simulink model "GridFormingConverter"  (R2024b)
settings: Solver=ode1be  StartTime=0.0  StopTime=simulationTime  FixedStep=gridInverter.vsm.samplingTime  MaxStep=gridInverter.vsm.samplingTime  RelTol=1e-3  AbsTol=1e-3
PreLoadFcn:
  | % Parameterize the model
  | GridFormingConverterInputParameters;
  | GFLParameters;
PostLoadFcn:
  | GridFormingConverterTestCondition;
  | GFLParameters;
undefined symbols (not defined in the file or in its folder): base, ConvCtrl, ConvPlt, DiscIntNeverNeededParam, Discrete, Fault, gcbh, GFMGFLSelect, grid, gridInverter, HMI, localSolverSampleTime, magnitude, PlantSim, scrFactorRg, scrFactorXg, sps, sps_rtmsupport, spsPLL3phModel, transformer, TransmissionLine, Trf
libraries: powerlib_extras x39, ee_lib x21, eeGeneralControl x19, nesl_utility x16, simulink x13, eeTransforms x10, fl_lib x7, spsSecondOrderFilterLib x4, spsabctodq0Lib x4, spsPower3phInstantaneousLib x3, spsMeanLib x2, eeSinGeneratorThreePhase x1
(part 3 of 6)

== system GridFormingConverter/BusCalculations/Measurement Unit (Phasor Computation)/Discrete Fourier(A) ==
  note: Discrete Fourier
  note: Pierre Giroux, Gilbert Sybille
      | Power System Simulation Laboratory
      | IREQ, Hydro-Quebc
  In : Inport
  Demux : Demux  Outputs=2
      settings: DisplayOption=none
  Discrete Mean value1 : powerlib_extras/Discrete Measurements/Discrete  Mean value  Freq=Freq  Vinit=Real_Init  Ts=Ts
  Discrete Mean value2 : powerlib_extras/Discrete Measurements/Discrete  Mean value  Freq=Freq  Vinit=Imag_Init  Ts=Ts
  Gain : Gain  Gain=2*pi*n*Freq  SaturateOnIntegerOverflow=on  OutDataTypeStr=Inherit: Same as input  ParamDataTypeStr=Inherit: Same as input
  Gain1 : Gain  Gain=k  SaturateOnIntegerOverflow=on  OutDataTypeStr=Inherit: Same as input  ParamDataTypeStr=Inherit: Same as input
  Mux : Mux  Inputs=2
  Product : Product  InputSameDT=on  SaturateOnIntegerOverflow=on  OutDataTypeStr=Inherit: Same as first input
  Real-Imag to Complex : RealImagToComplex
  Trigonometric Function : Trigonometry
  Trigonometric Function1 : Trigonometry  Operator=cos
  t : DigitalClock  SampleTime=Ts
  Fund : Outport
  wires:
  Real-Imag to Complex/1 -> Fund/1
  Discrete Mean value2/1 -> Real-Imag to Complex/2  "Imag"
  Discrete Mean value1/1 -> Real-Imag to Complex/1  "Real"
  t/1 -> Gain/1
  Gain/1 -> Trigonometric Function/1, Trigonometric Function1/1
  Trigonometric Function/1 -> Mux/1
  Trigonometric Function1/1 -> Mux/2
  Mux/1 -> Gain1/1
  In/1 -> Product/1
  Gain1/1 -> Product/2
  Product/1 -> Demux/1
  Demux/1 -> Discrete Mean value1/1
  Demux/2 -> Discrete Mean value2/1

== system GridFormingConverter/BusCalculations/Measurement Unit (Phasor Computation)/Discrete Fourier(A)  ==
  note: Pierre Giroux, Gilbert Sybille
      | Power System Simulation Laboratory
      | IREQ, Hydro-Quebc
  note: Discrete Fourier
  In : Inport
  Demux : Demux  Outputs=2
      settings: DisplayOption=none
  Discrete Mean value1 : powerlib_extras/Discrete Measurements/Discrete  Mean value  Freq=Freq  Vinit=Real_Init  Ts=Ts
  Discrete Mean value2 : powerlib_extras/Discrete Measurements/Discrete  Mean value  Freq=Freq  Vinit=Imag_Init  Ts=Ts
  Gain : Gain  Gain=2*pi*n*Freq  SaturateOnIntegerOverflow=on  OutDataTypeStr=Inherit: Same as input  ParamDataTypeStr=Inherit: Same as input
  Gain1 : Gain  Gain=k  SaturateOnIntegerOverflow=on  OutDataTypeStr=Inherit: Same as input  ParamDataTypeStr=Inherit: Same as input
  Mux : Mux  Inputs=2
  Product : Product  InputSameDT=on  SaturateOnIntegerOverflow=on  OutDataTypeStr=Inherit: Same as first input
  Real-Imag to Complex : RealImagToComplex
  Trigonometric Function : Trigonometry
  Trigonometric Function1 : Trigonometry  Operator=cos
  t : DigitalClock  SampleTime=Ts
  Fund : Outport
  wires:
  Demux/2 -> Discrete Mean value2/1
  Demux/1 -> Discrete Mean value1/1
  Product/1 -> Demux/1
  Gain1/1 -> Product/2
  In/1 -> Product/1
  Mux/1 -> Gain1/1
  Trigonometric Function1/1 -> Mux/2
  Trigonometric Function/1 -> Mux/1
  Gain/1 -> Trigonometric Function1/1, Trigonometric Function/1
  t/1 -> Gain/1
  Discrete Mean value1/1 -> Real-Imag to Complex/1  "Real"
  Discrete Mean value2/1 -> Real-Imag to Complex/2  "Imag"
  Real-Imag to Complex/1 -> Fund/1

== system GridFormingConverter/BusCalculations/Measurement Unit (Phasor Computation)/Discrete Fourier(B) ==
  note: Pierre Giroux, Gilbert Sybille
      | Power System Simulation Laboratory
      | IREQ, Hydro-Quebc
  note: Discrete Fourier
  In : Inport
  Demux : Demux  Outputs=2
      settings: DisplayOption=none
  Discrete Mean value1 : powerlib_extras/Discrete Measurements/Discrete  Mean value  Freq=Freq  Vinit=Real_Init  Ts=Ts
  Discrete Mean value2 : powerlib_extras/Discrete Measurements/Discrete  Mean value  Freq=Freq  Vinit=Imag_Init  Ts=Ts
  Gain : Gain  Gain=2*pi*n*Freq  SaturateOnIntegerOverflow=on  OutDataTypeStr=Inherit: Same as input  ParamDataTypeStr=Inherit: Same as input
  Gain1 : Gain  Gain=k  SaturateOnIntegerOverflow=on  OutDataTypeStr=Inherit: Same as input  ParamDataTypeStr=Inherit: Same as input
  Mux : Mux  Inputs=2
  Product : Product  InputSameDT=on  SaturateOnIntegerOverflow=on  OutDataTypeStr=Inherit: Same as first input
  Real-Imag to Complex : RealImagToComplex
  Trigonometric Function : Trigonometry
  Trigonometric Function1 : Trigonometry  Operator=cos
  t : DigitalClock  SampleTime=Ts
  Fund : Outport
  wires:
  Demux/2 -> Discrete Mean value2/1
  Demux/1 -> Discrete Mean value1/1
  Product/1 -> Demux/1
  Gain1/1 -> Product/2
  In/1 -> Product/1
  Mux/1 -> Gain1/1
  Trigonometric Function1/1 -> Mux/2
  Trigonometric Function/1 -> Mux/1
  Gain/1 -> Trigonometric Function1/1, Trigonometric Function/1
  t/1 -> Gain/1
  Discrete Mean value1/1 -> Real-Imag to Complex/1  "Real"
  Discrete Mean value2/1 -> Real-Imag to Complex/2  "Imag"
  Real-Imag to Complex/1 -> Fund/1

== system GridFormingConverter/BusCalculations/Measurement Unit (Phasor Computation)/Discrete Fourier(B)  ==
  note: Discrete Fourier
  note: Pierre Giroux, Gilbert Sybille
      | Power System Simulation Laboratory
      | IREQ, Hydro-Quebc
  In : Inport
  Demux : Demux  Outputs=2
      settings: DisplayOption=none
  Discrete Mean value1 : powerlib_extras/Discrete Measurements/Discrete  Mean value  Freq=Freq  Vinit=Real_Init  Ts=Ts
  Discrete Mean value2 : powerlib_extras/Discrete Measurements/Discrete  Mean value  Freq=Freq  Vinit=Imag_Init  Ts=Ts
  Gain : Gain  Gain=2*pi*n*Freq  SaturateOnIntegerOverflow=on  OutDataTypeStr=Inherit: Same as input  ParamDataTypeStr=Inherit: Same as input
  Gain1 : Gain  Gain=k  SaturateOnIntegerOverflow=on  OutDataTypeStr=Inherit: Same as input  ParamDataTypeStr=Inherit: Same as input
  Mux : Mux  Inputs=2
  Product : Product  InputSameDT=on  SaturateOnIntegerOverflow=on  OutDataTypeStr=Inherit: Same as first input
  Real-Imag to Complex : RealImagToComplex
  Trigonometric Function : Trigonometry
  Trigonometric Function1 : Trigonometry  Operator=cos
  t : DigitalClock  SampleTime=Ts
  Fund : Outport
  wires:
  Real-Imag to Complex/1 -> Fund/1
  Discrete Mean value2/1 -> Real-Imag to Complex/2  "Imag"
  Discrete Mean value1/1 -> Real-Imag to Complex/1  "Real"
  t/1 -> Gain/1
  Gain/1 -> Trigonometric Function/1, Trigonometric Function1/1
  Trigonometric Function/1 -> Mux/1
  Trigonometric Function1/1 -> Mux/2
  Mux/1 -> Gain1/1
  In/1 -> Product/1
  Gain1/1 -> Product/2
  Product/1 -> Demux/1
  Demux/1 -> Discrete Mean value1/1
  Demux/2 -> Discrete Mean value2/1

== system GridFormingConverter/BusCalculations/Measurement Unit (Phasor Computation)/Discrete Fourier(C) ==
  note: Discrete Fourier
  note: Pierre Giroux, Gilbert Sybille
      | Power System Simulation Laboratory
      | IREQ, Hydro-Quebc
  In : Inport
  Demux : Demux  Outputs=2
      settings: DisplayOption=none
  Discrete Mean value1 : powerlib_extras/Discrete Measurements/Discrete  Mean value  Freq=Freq  Vinit=Real_Init  Ts=Ts
  Discrete Mean value2 : powerlib_extras/Discrete Measurements/Discrete  Mean value  Freq=Freq  Vinit=Imag_Init  Ts=Ts
  Gain : Gain  Gain=2*pi*n*Freq  SaturateOnIntegerOverflow=on  OutDataTypeStr=Inherit: Same as input  ParamDataTypeStr=Inherit: Same as input
  Gain1 : Gain  Gain=k  SaturateOnIntegerOverflow=on  OutDataTypeStr=Inherit: Same as input  ParamDataTypeStr=Inherit: Same as input
  Mux : Mux  Inputs=2
  Product : Product  InputSameDT=on  SaturateOnIntegerOverflow=on  OutDataTypeStr=Inherit: Same as first input
  Real-Imag to Complex : RealImagToComplex
  Trigonometric Function : Trigonometry
  Trigonometric Function1 : Trigonometry  Operator=cos
  t : DigitalClock  SampleTime=Ts
  Fund : Outport
  wires:
  Real-Imag to Complex/1 -> Fund/1
  Discrete Mean value2/1 -> Real-Imag to Complex/2  "Imag"
  Discrete Mean value1/1 -> Real-Imag to Complex/1  "Real"
  t/1 -> Gain/1
  Gain/1 -> Trigonometric Function/1, Trigonometric Function1/1
  Trigonometric Function/1 -> Mux/1
  Trigonometric Function1/1 -> Mux/2
  Mux/1 -> Gain1/1
  In/1 -> Product/1
  Gain1/1 -> Product/2
  Product/1 -> Demux/1
  Demux/1 -> Discrete Mean value1/1
  Demux/2 -> Discrete Mean value2/1

== system GridFormingConverter/BusCalculations/Measurement Unit (Phasor Computation)/Discrete Fourier(C)  ==
  note: Pierre Giroux, Gilbert Sybille
      | Power System Simulation Laboratory
      | IREQ, Hydro-Quebc
  note: Discrete Fourier
  In : Inport
  Demux : Demux  Outputs=2
      settings: DisplayOption=none
  Discrete Mean value1 : powerlib_extras/Discrete Measurements/Discrete  Mean value  Freq=Freq  Vinit=Real_Init  Ts=Ts
  Discrete Mean value2 : powerlib_extras/Discrete Measurements/Discrete  Mean value  Freq=Freq  Vinit=Imag_Init  Ts=Ts
  Gain : Gain  Gain=2*pi*n*Freq  SaturateOnIntegerOverflow=on  OutDataTypeStr=Inherit: Same as input  ParamDataTypeStr=Inherit: Same as input
  Gain1 : Gain  Gain=k  SaturateOnIntegerOverflow=on  OutDataTypeStr=Inherit: Same as input  ParamDataTypeStr=Inherit: Same as input
  Mux : Mux  Inputs=2
  Product : Product  InputSameDT=on  SaturateOnIntegerOverflow=on  OutDataTypeStr=Inherit: Same as first input
  Real-Imag to Complex : RealImagToComplex
  Trigonometric Function : Trigonometry
  Trigonometric Function1 : Trigonometry  Operator=cos
  t : DigitalClock  SampleTime=Ts
  Fund : Outport
  wires:
  Demux/2 -> Discrete Mean value2/1
  Demux/1 -> Discrete Mean value1/1
  Product/1 -> Demux/1
  Gain1/1 -> Product/2
  In/1 -> Product/1
  Mux/1 -> Gain1/1
  Trigonometric Function1/1 -> Mux/2
  Trigonometric Function/1 -> Mux/1
  Gain/1 -> Trigonometric Function1/1, Trigonometric Function/1
  t/1 -> Gain/1
  Discrete Mean value1/1 -> Real-Imag to Complex/1  "Real"
  Discrete Mean value2/1 -> Real-Imag to Complex/2  "Imag"
  Real-Imag to Complex/1 -> Fund/1

== system GridFormingConverter/BusCalculations1/Measurement Unit (Phasor Computation)/Discrete Fourier(A) ==
  note: Pierre Giroux, Gilbert Sybille
      | Power System Simulation Laboratory
      | IREQ, Hydro-Quebc
  note: Discrete Fourier
  In : Inport
  Demux : Demux  Outputs=2
      settings: DisplayOption=none
  Discrete Mean value1 : powerlib_extras/Discrete Measurements/Discrete  Mean value  Freq=Freq  Vinit=Real_Init  Ts=Ts
  Discrete Mean value2 : powerlib_extras/Discrete Measurements/Discrete  Mean value  Freq=Freq  Vinit=Imag_Init  Ts=Ts
  Gain : Gain  Gain=2*pi*n*Freq  SaturateOnIntegerOverflow=on  OutDataTypeStr=Inherit: Same as input  ParamDataTypeStr=Inherit: Same as input
  Gain1 : Gain  Gain=k  SaturateOnIntegerOverflow=on  OutDataTypeStr=Inherit: Same as input  ParamDataTypeStr=Inherit: Same as input
  Mux : Mux  Inputs=2
  Product : Product  InputSameDT=on  SaturateOnIntegerOverflow=on  OutDataTypeStr=Inherit: Same as first input
  Real-Imag to Complex : RealImagToComplex
  Trigonometric Function : Trigonometry
  Trigonometric Function1 : Trigonometry  Operator=cos
  t : DigitalClock  SampleTime=Ts
  Fund : Outport
  wires:
  Demux/2 -> Discrete Mean value2/1
  Demux/1 -> Discrete Mean value1/1
  Product/1 -> Demux/1
  Gain1/1 -> Product/2
  In/1 -> Product/1
  Mux/1 -> Gain1/1
  Trigonometric Function1/1 -> Mux/2
  Trigonometric Function/1 -> Mux/1
  Gain/1 -> Trigonometric Function1/1, Trigonometric Function/1
  t/1 -> Gain/1
  Discrete Mean value1/1 -> Real-Imag to Complex/1  "Real"
  Discrete Mean value2/1 -> Real-Imag to Complex/2  "Imag"
  Real-Imag to Complex/1 -> Fund/1

== system GridFormingConverter/BusCalculations1/Measurement Unit (Phasor Computation)/Discrete Fourier(A)  ==
  note: Discrete Fourier
  note: Pierre Giroux, Gilbert Sybille
      | Power System Simulation Laboratory
      | IREQ, Hydro-Quebc
  In : Inport
  Demux : Demux  Outputs=2
      settings: DisplayOption=none
  Discrete Mean value1 : powerlib_extras/Discrete Measurements/Discrete  Mean value  Freq=Freq  Vinit=Real_Init  Ts=Ts
  Discrete Mean value2 : powerlib_extras/Discrete Measurements/Discrete  Mean value  Freq=Freq  Vinit=Imag_Init  Ts=Ts
  Gain : Gain  Gain=2*pi*n*Freq  SaturateOnIntegerOverflow=on  OutDataTypeStr=Inherit: Same as input  ParamDataTypeStr=Inherit: Same as input
  Gain1 : Gain  Gain=k  SaturateOnIntegerOverflow=on  OutDataTypeStr=Inherit: Same as input  ParamDataTypeStr=Inherit: Same as input
  Mux : Mux  Inputs=2
  Product : Product  InputSameDT=on  SaturateOnIntegerOverflow=on  OutDataTypeStr=Inherit: Same as first input
  Real-Imag to Complex : RealImagToComplex
  Trigonometric Function : Trigonometry
  Trigonometric Function1 : Trigonometry  Operator=cos
  t : DigitalClock  SampleTime=Ts
  Fund : Outport
  wires:
  Real-Imag to Complex/1 -> Fund/1
  Discrete Mean value2/1 -> Real-Imag to Complex/2  "Imag"
  Discrete Mean value1/1 -> Real-Imag to Complex/1  "Real"
  t/1 -> Gain/1
  Gain/1 -> Trigonometric Function/1, Trigonometric Function1/1
  Trigonometric Function/1 -> Mux/1
  Trigonometric Function1/1 -> Mux/2
  Mux/1 -> Gain1/1
  In/1 -> Product/1
  Gain1/1 -> Product/2
  Product/1 -> Demux/1
  Demux/1 -> Discrete Mean value1/1
  Demux/2 -> Discrete Mean value2/1

== system GridFormingConverter/BusCalculations1/Measurement Unit (Phasor Computation)/Discrete Fourier(B) ==
  note: Discrete Fourier
  note: Pierre Giroux, Gilbert Sybille
      | Power System Simulation Laboratory
      | IREQ, Hydro-Quebc
  In : Inport
  Demux : Demux  Outputs=2
      settings: DisplayOption=none
  Discrete Mean value1 : powerlib_extras/Discrete Measurements/Discrete  Mean value  Freq=Freq  Vinit=Real_Init  Ts=Ts
  Discrete Mean value2 : powerlib_extras/Discrete Measurements/Discrete  Mean value  Freq=Freq  Vinit=Imag_Init  Ts=Ts
  Gain : Gain  Gain=2*pi*n*Freq  SaturateOnIntegerOverflow=on  OutDataTypeStr=Inherit: Same as input  ParamDataTypeStr=Inherit: Same as input
  Gain1 : Gain  Gain=k  SaturateOnIntegerOverflow=on  OutDataTypeStr=Inherit: Same as input  ParamDataTypeStr=Inherit: Same as input
  Mux : Mux  Inputs=2
  Product : Product  InputSameDT=on  SaturateOnIntegerOverflow=on  OutDataTypeStr=Inherit: Same as first input
  Real-Imag to Complex : RealImagToComplex
  Trigonometric Function : Trigonometry
  Trigonometric Function1 : Trigonometry  Operator=cos
  t : DigitalClock  SampleTime=Ts
  Fund : Outport
  wires:
  Real-Imag to Complex/1 -> Fund/1
  Discrete Mean value2/1 -> Real-Imag to Complex/2  "Imag"
  Discrete Mean value1/1 -> Real-Imag to Complex/1  "Real"
  t/1 -> Gain/1
  Gain/1 -> Trigonometric Function/1, Trigonometric Function1/1
  Trigonometric Function/1 -> Mux/1
  Trigonometric Function1/1 -> Mux/2
  Mux/1 -> Gain1/1
  In/1 -> Product/1
  Gain1/1 -> Product/2
  Product/1 -> Demux/1
  Demux/1 -> Discrete Mean value1/1
  Demux/2 -> Discrete Mean value2/1

== system GridFormingConverter/BusCalculations1/Measurement Unit (Phasor Computation)/Discrete Fourier(B)  ==
  note: Pierre Giroux, Gilbert Sybille
      | Power System Simulation Laboratory
      | IREQ, Hydro-Quebc
  note: Discrete Fourier
  In : Inport
  Demux : Demux  Outputs=2
      settings: DisplayOption=none
  Discrete Mean value1 : powerlib_extras/Discrete Measurements/Discrete  Mean value  Freq=Freq  Vinit=Real_Init  Ts=Ts
  Discrete Mean value2 : powerlib_extras/Discrete Measurements/Discrete  Mean value  Freq=Freq  Vinit=Imag_Init  Ts=Ts
  Gain : Gain  Gain=2*pi*n*Freq  SaturateOnIntegerOverflow=on  OutDataTypeStr=Inherit: Same as input  ParamDataTypeStr=Inherit: Same as input
  Gain1 : Gain  Gain=k  SaturateOnIntegerOverflow=on  OutDataTypeStr=Inherit: Same as input  ParamDataTypeStr=Inherit: Same as input
  Mux : Mux  Inputs=2
  Product : Product  InputSameDT=on  SaturateOnIntegerOverflow=on  OutDataTypeStr=Inherit: Same as first input
  Real-Imag to Complex : RealImagToComplex
  Trigonometric Function : Trigonometry
  Trigonometric Function1 : Trigonometry  Operator=cos
  t : DigitalClock  SampleTime=Ts
  Fund : Outport
  wires:
  Demux/2 -> Discrete Mean value2/1
  Demux/1 -> Discrete Mean value1/1
  Product/1 -> Demux/1
  Gain1/1 -> Product/2
  In/1 -> Product/1
  Mux/1 -> Gain1/1
  Trigonometric Function1/1 -> Mux/2
  Trigonometric Function/1 -> Mux/1
  Gain/1 -> Trigonometric Function1/1, Trigonometric Function/1
  t/1 -> Gain/1
  Discrete Mean value1/1 -> Real-Imag to Complex/1  "Real"
  Discrete Mean value2/1 -> Real-Imag to Complex/2  "Imag"
  Real-Imag to Complex/1 -> Fund/1

== system GridFormingConverter/BusCalculations1/Measurement Unit (Phasor Computation)/Discrete Fourier(C) ==
  note: Pierre Giroux, Gilbert Sybille
      | Power System Simulation Laboratory
      | IREQ, Hydro-Quebc
  note: Discrete Fourier
  In : Inport
  Demux : Demux  Outputs=2
      settings: DisplayOption=none
  Discrete Mean value1 : powerlib_extras/Discrete Measurements/Discrete  Mean value  Freq=Freq  Vinit=Real_Init  Ts=Ts
  Discrete Mean value2 : powerlib_extras/Discrete Measurements/Discrete  Mean value  Freq=Freq  Vinit=Imag_Init  Ts=Ts
  Gain : Gain  Gain=2*pi*n*Freq  SaturateOnIntegerOverflow=on  OutDataTypeStr=Inherit: Same as input  ParamDataTypeStr=Inherit: Same as input
  Gain1 : Gain  Gain=k  SaturateOnIntegerOverflow=on  OutDataTypeStr=Inherit: Same as input  ParamDataTypeStr=Inherit: Same as input
  Mux : Mux  Inputs=2
  Product : Product  InputSameDT=on  SaturateOnIntegerOverflow=on  OutDataTypeStr=Inherit: Same as first input
  Real-Imag to Complex : RealImagToComplex
  Trigonometric Function : Trigonometry
  Trigonometric Function1 : Trigonometry  Operator=cos
  t : DigitalClock  SampleTime=Ts
  Fund : Outport
  wires:
  Demux/2 -> Discrete Mean value2/1
  Demux/1 -> Discrete Mean value1/1
  Product/1 -> Demux/1
  Gain1/1 -> Product/2
  In/1 -> Product/1
  Mux/1 -> Gain1/1
  Trigonometric Function1/1 -> Mux/2
  Trigonometric Function/1 -> Mux/1
  Gain/1 -> Trigonometric Function1/1, Trigonometric Function/1
  t/1 -> Gain/1
  Discrete Mean value1/1 -> Real-Imag to Complex/1  "Real"
  Discrete Mean value2/1 -> Real-Imag to Complex/2  "Imag"
  Real-Imag to Complex/1 -> Fund/1

== system GridFormingConverter/BusCalculations1/Measurement Unit (Phasor Computation)/Discrete Fourier(C)  ==
  note: Discrete Fourier
  note: Pierre Giroux, Gilbert Sybille
      | Power System Simulation Laboratory
      | IREQ, Hydro-Quebc
  In : Inport
  Demux : Demux  Outputs=2
      settings: DisplayOption=none
  Discrete Mean value1 : powerlib_extras/Discrete Measurements/Discrete  Mean value  Freq=Freq  Vinit=Real_Init  Ts=Ts
  Discrete Mean value2 : powerlib_extras/Discrete Measurements/Discrete  Mean value  Freq=Freq  Vinit=Imag_Init  Ts=Ts
  Gain : Gain  Gain=2*pi*n*Freq  SaturateOnIntegerOverflow=on  OutDataTypeStr=Inherit: Same as input  ParamDataTypeStr=Inherit: Same as input
  Gain1 : Gain  Gain=k  SaturateOnIntegerOverflow=on  OutDataTypeStr=Inherit: Same as input  ParamDataTypeStr=Inherit: Same as input
  Mux : Mux  Inputs=2
  Product : Product  InputSameDT=on  SaturateOnIntegerOverflow=on  OutDataTypeStr=Inherit: Same as first input
  Real-Imag to Complex : RealImagToComplex
  Trigonometric Function : Trigonometry
  Trigonometric Function1 : Trigonometry  Operator=cos
  t : DigitalClock  SampleTime=Ts
  Fund : Outport
  wires:
  Real-Imag to Complex/1 -> Fund/1
  Discrete Mean value2/1 -> Real-Imag to Complex/2  "Imag"
  Discrete Mean value1/1 -> Real-Imag to Complex/1  "Real"
  t/1 -> Gain/1
  Gain/1 -> Trigonometric Function/1, Trigonometric Function1/1
  Trigonometric Function/1 -> Mux/1
  Trigonometric Function1/1 -> Mux/2
  Mux/1 -> Gain1/1
  In/1 -> Product/1
  Gain1/1 -> Product/2
  Product/1 -> Demux/1
  Demux/1 -> Discrete Mean value1/1
  Demux/2 -> Discrete Mean value2/1

== system GridFormingConverter/Grid-Forming Converter/BusCalculations/Complex2Phasor ==
  complex : Inport
  Bus Creator1 : BusCreator  Inputs=3
  Bus Creator2 : BusCreator  Inputs=2
  Bus Creator3 : BusCreator  Inputs=2
  Bus Creator5 : BusCreator  Inputs=2
  Complex to Magnitude-Angle3 : ComplexToMagnitudeAngle
  Demux2 : Demux  Outputs=3
  Demux3 : Demux  Outputs=3
  Gain : Gain  Gain=180/pi
  Phasor : Outport
  wires:
  complex/1 -> Complex to Magnitude-Angle3/1
  Demux2/3 -> Bus Creator3/1  "mag"
  Complex to Magnitude-Angle3/1 -> Demux2/1
  Demux3/2 -> Bus Creator5/2  "phase"
  Demux2/1 -> Bus Creator2/1  "mag"
  Complex to Magnitude-Angle3/2 -> Gain/1
  Demux2/2 -> Bus Creator5/1  "mag"
  Demux3/1 -> Bus Creator2/2  "phase"
  Demux3/3 -> Bus Creator3/2  "phase"
  Bus Creator2/1 -> Bus Creator1/1  "a"
  Bus Creator5/1 -> Bus Creator1/2  "b"
  Bus Creator3/1 -> Bus Creator1/3  "c"
  Bus Creator1/1 -> Phasor/1  "Phasor"
  Gain/1 -> Demux3/1

== system GridFormingConverter/Grid-Forming Converter/BusCalculations/Complex2Phasor1 ==
  complex : Inport
  Bus Creator1 : BusCreator  Inputs=3
  Bus Creator2 : BusCreator  Inputs=2
  Bus Creator3 : BusCreator  Inputs=2
  Bus Creator5 : BusCreator  Inputs=2
  Complex to Magnitude-Angle3 : ComplexToMagnitudeAngle
  Demux2 : Demux  Outputs=3
  Demux3 : Demux  Outputs=3
  Gain : Gain  Gain=180/pi
  Phasor : Outport
  wires:
  Bus Creator1/1 -> Phasor/1  "Phasor"
  Bus Creator3/1 -> Bus Creator1/3  "c"
  Bus Creator5/1 -> Bus Creator1/2  "b"
  Bus Creator2/1 -> Bus Creator1/1  "a"
  Demux3/3 -> Bus Creator3/2  "phase"
  Demux3/1 -> Bus Creator2/2  "phase"
  Demux2/2 -> Bus Creator5/1  "mag"
  Complex to Magnitude-Angle3/2 -> Gain/1
  Demux2/1 -> Bus Creator2/1  "mag"
  Demux3/2 -> Bus Creator5/2  "phase"
  Complex to Magnitude-Angle3/1 -> Demux2/1
  Demux2/3 -> Bus Creator3/1  "mag"
  complex/1 -> Complex to Magnitude-Angle3/1
  Gain/1 -> Demux3/1

== system GridFormingConverter/Grid-Forming Converter/BusCalculations/Measurement Unit (Phasor Computation) ==
  Vabc(t) : Inport  PortDimensions=3
  Iabc(t) : Inport  Port=2  PortDimensions=3
  Demux : Demux  Outputs=3
      settings: DisplayOption=none
  Demux1 : Demux  Outputs=3
      settings: DisplayOption=none
  Discrete Fourier(A) : Subsystem  AncestorBlock=|  mask(Discrete Fourier){Freq=Freq, n=1, Par_Init=[0 0], Ts=Ts}
      | powerlib_extras/Discrete
      | Measurements/Discrete 
      | Fourier
      mask prompts: Freq "Fundamental frequency (Hz):"; n "Harmonic n (0=DC; 1=fundamental; 2=2nd harm;  ...):"; Par_Init "Initial input: [ Mag  Phase(degrees) ]"; Ts "Sample time:"
      mask help:
      | This block computes the fundamental value of the input signal over a running window of one cycle of the specified fundamental frequency. First and second outputs return respectively the magnitude and phase (degrees) of the fundamental.
      | For the first cycle of simulation, the ouputs are held constant to the value specified by the parameter "Initial input".
      mask init: same as GridFormingConverter/BusCalculations/Measurement Unit (Phasor Computation)/Discrete Fourier(A)
  "Discrete Fourier(A) " : Subsystem  AncestorBlock=|  mask(Discrete Fourier){Freq=Freq, n=1, Par_Init=[0 0], Ts=Ts}
      | powerlib_extras/Discrete
      | Measurements/Discrete 
      | Fourier
      mask prompts: Freq "Fundamental frequency (Hz):"; n "Harmonic n (0=DC; 1=fundamental; 2=2nd harm;  ...):"; Par_Init "Initial input: [ Mag  Phase(degrees) ]"; Ts "Sample time:"
      mask help:
      | This block computes the fundamental value of the input signal over a running window of one cycle of the specified fundamental frequency. First and second outputs return respectively the magnitude and phase (degrees) of the fundamental.
      | For the first cycle of simulation, the ouputs are held constant to the value specified by the parameter "Initial input".
      mask init: same as GridFormingConverter/BusCalculations/Measurement Unit (Phasor Computation)/Discrete Fourier(A)
  Discrete Fourier(B) : Subsystem  AncestorBlock=|  mask(Discrete Fourier){Freq=Freq, n=1, Par_Init=[0 -120], Ts=Ts}
      | powerlib_extras/Discrete
      | Measurements/Discrete 
      | Fourier
      mask prompts: Freq "Fundamental frequency (Hz):"; n "Harmonic n (0=DC; 1=fundamental; 2=2nd harm;  ...):"; Par_Init "Initial input: [ Mag  Phase(degrees) ]"; Ts "Sample time:"
      mask help:
      | This block computes the fundamental value of the input signal over a running window of one cycle of the specified fundamental frequency. First and second outputs return respectively the magnitude and phase (degrees) of the fundamental.
      | For the first cycle of simulation, the ouputs are held constant to the value specified by the parameter "Initial input".
      mask init: same as GridFormingConverter/BusCalculations/Measurement Unit (Phasor Computation)/Discrete Fourier(A)
  "Discrete Fourier(B) " : Subsystem  AncestorBlock=|  mask(Discrete Fourier){Freq=Freq, n=1, Par_Init=[0 -120], Ts=Ts}
      | powerlib_extras/Discrete
      | Measurements/Discrete 
      | Fourier
      mask prompts: Freq "Fundamental frequency (Hz):"; n "Harmonic n (0=DC; 1=fundamental; 2=2nd harm;  ...):"; Par_Init "Initial input: [ Mag  Phase(degrees) ]"; Ts "Sample time:"
      mask help:
      | This block computes the fundamental value of the input signal over a running window of one cycle of the specified fundamental frequency. First and second outputs return respectively the magnitude and phase (degrees) of the fundamental.
      | For the first cycle of simulation, the ouputs are held constant to the value specified by the parameter "Initial input".
      mask init: same as GridFormingConverter/BusCalculations/Measurement Unit (Phasor Computation)/Discrete Fourier(A)
  Discrete Fourier(C) : Subsystem  AncestorBlock=|  mask(Discrete Fourier){Freq=Freq, n=1, Par_Init=[0 120], Ts=Ts}
      | powerlib_extras/Discrete
      | Measurements/Discrete 
      | Fourier
      mask prompts: Freq "Fundamental frequency (Hz):"; n "Harmonic n (0=DC; 1=fundamental; 2=2nd harm;  ...):"; Par_Init "Initial input: [ Mag  Phase(degrees) ]"; Ts "Sample time:"
      mask help:
      | This block computes the fundamental value of the input signal over a running window of one cycle of the specified fundamental frequency. First and second outputs return respectively the magnitude and phase (degrees) of the fundamental.
      | For the first cycle of simulation, the ouputs are held constant to the value specified by the parameter "Initial input".
      mask init: same as GridFormingConverter/BusCalculations/Measurement Unit (Phasor Computation)/Discrete Fourier(A)
  "Discrete Fourier(C) " : Subsystem  AncestorBlock=|  mask(Discrete Fourier){Freq=Freq, n=1, Par_Init=[0 120], Ts=Ts}
      | powerlib_extras/Discrete
      | Measurements/Discrete 
      | Fourier
      mask prompts: Freq "Fundamental frequency (Hz):"; n "Harmonic n (0=DC; 1=fundamental; 2=2nd harm;  ...):"; Par_Init "Initial input: [ Mag  Phase(degrees) ]"; Ts "Sample time:"
      mask help:
      | This block computes the fundamental value of the input signal over a running window of one cycle of the specified fundamental frequency. First and second outputs return respectively the magnitude and phase (degrees) of the fundamental.
      | For the first cycle of simulation, the ouputs are held constant to the value specified by the parameter "Initial input".
      mask init: same as GridFormingConverter/BusCalculations/Measurement Unit (Phasor Computation)/Discrete Fourier(A)
  Mux : Mux  Inputs=3
  Mux1 : Mux  Inputs=3
  Vabc_Fund : Outport
  " Iabc_Fund" : Outport  Port=2
  wires:
  "Discrete Fourier(C) "/1(Fund) -> Mux1/3
  "Discrete Fourier(B) "/1(Fund) -> Mux1/2
  "Discrete Fourier(A) "/1(Fund) -> Mux1/1
  Mux1/1 -> " Iabc_Fund"/1
  Iabc(t)/1 -> Demux1/1
  Demux1/3 -> "Discrete Fourier(C) "/1(In)
  Demux1/2 -> "Discrete Fourier(B) "/1(In)
  Demux1/1 -> "Discrete Fourier(A) "/1(In)
  Mux/1 -> Vabc_Fund/1
  Discrete Fourier(C)/1(Fund) -> Mux/3
  Discrete Fourier(B)/1(Fund) -> Mux/2
  Discrete Fourier(A)/1(Fund) -> Mux/1
  Demux/3 -> Discrete Fourier(C)/1(In)
  Demux/2 -> Discrete Fourier(B)/1(In)
  Vabc(t)/1 -> Demux/1
  Demux/1 -> Discrete Fourier(A)/1(In)

== system GridFormingConverter/Grid-Forming Converter/BusCalculations/SymmetricalComponentsCalc ==
  abc : Inport
  Bus Creator{,1..4,7..8} (7 alike) : BusCreator  Inputs=3
  Bus Creator5 : BusCreator  Inputs=2
  Bus Creator6 : BusCreator  Inputs=2
  Bus Creator9 : BusCreator  Inputs=2
  Complex to Magnitude-Angle1 : ComplexToMagnitudeAngle
  Complex to Magnitude-Angle2 : ComplexToMagnitudeAngle
  Complex to Magnitude-Angle3 : ComplexToMagnitudeAngle
  Demux{,1..5} (6 alike) : Demux  Outputs=3
  Gain : Gain  Gain=[exp(1i*4*pi/3) 0 0; 0 exp(1i*2*pi/3) 0; 0 0 1]  Multiplication=Matrix(K*u)
  Gain1 : Gain  Gain=[exp(1i*2*pi/3) 0 0; 0 exp(1i*4*pi/3) 0; 0 0 1]  Multiplication=Matrix(K*u)
  Gain2 : Gain  Gain=180/pi
  Gain3 : Gain  Gain=180/pi
  Gain4 : Gain  Gain=180/pi
  Symmetrical-Components Transform1 : eeTransforms/Symmetrical-Components Transform  PowerInvariant=off
  ABC+-0 : Outport
  wires:
  Demux/2 -> Bus Creator3/2  "neg"
  Complex to Magnitude-Angle3/2 -> Gain2/1
  Demux/1 -> Bus Creator3/1  "pos"
  Symmetrical-Components Transform1/1 -> Complex to Magnitude-Angle3/1, Gain/1, Gain1/1
  Demux/3 -> Bus Creator3/3  "zero"
  Bus Creator3/1 -> Bus Creator5/1  "mag"
  Complex to Magnitude-Angle3/1 -> Demux/1
  Bus Creator4/1 -> Bus Creator5/2  "phase"
  abc/1 -> Symmetrical-Components Transform1/1
  Bus Creator5/1 -> Bus Creator/1  "A"
  Bus Creator6/1 -> Bus Creator/2  "B"
  Bus Creator2/1 -> Bus Creator6/2  "phase"
  Complex to Magnitude-Angle1/1 -> Demux2/1
  Bus Creator1/1 -> Bus Creator6/1  "mag"
  Complex to Magnitude-Angle1/2 -> Gain3/1
  Gain/1 -> Complex to Magnitude-Angle1/1
  Complex to Magnitude-Angle2/2 -> Gain4/1
  Bus Creator7/1 -> Bus Creator9/1  "mag"
  Complex to Magnitude-Angle2/1 -> Demux4/1
  Bus Creator8/1 -> Bus Creator9/2  "phase"
  Bus Creator9/1 -> Bus Creator/3  "C"
  Gain1/1 -> Complex to Magnitude-Angle2/1
  Bus Creator/1 -> ABC+-0/1
  Demux1/1 -> Bus Creator4/1  "pos"
  Demux1/3 -> Bus Creator4/3  "zero"
  Demux1/2 -> Bus Creator4/2  "neg"
  Demux2/2 -> Bus Creator1/2  "neg"
  Demux2/3 -> Bus Creator1/3  "zero"
  Demux2/1 -> Bus Creator1/1  "pos"
  Demux3/2 -> Bus Creator2/2  "neg"
  Demux3/3 -> Bus Creator2/3  "zero"
  Demux3/1 -> Bus Creator2/1  "pos"
  Demux4/2 -> Bus Creator7/2  "neg"
  Demux4/3 -> Bus Creator7/3  "zero"
  Demux4/1 -> Bus Creator7/1  "pos"
  Demux5/2 -> Bus Creator8/2  "neg"
  Demux5/3 -> Bus Creator8/3  "zero"
  Demux5/1 -> Bus Creator8/1  "pos"
  Gain2/1 -> Demux1/1
  Gain3/1 -> Demux3/1
  Gain4/1 -> Demux5/1

== system GridFormingConverter/Grid-Forming Converter/BusCalculations/SymmetricalComponentsCalc1 ==
  abc : Inport
  Bus Creator{,1..4,7..8} (7 alike) : BusCreator  Inputs=3
  Bus Creator5 : BusCreator  Inputs=2
  Bus Creator6 : BusCreator  Inputs=2
  Bus Creator9 : BusCreator  Inputs=2
  Complex to Magnitude-Angle1 : ComplexToMagnitudeAngle
  Complex to Magnitude-Angle2 : ComplexToMagnitudeAngle
  Complex to Magnitude-Angle3 : ComplexToMagnitudeAngle
  Demux{,1..5} (6 alike) : Demux  Outputs=3
  Gain : Gain  Gain=[exp(1i*4*pi/3) 0 0; 0 exp(1i*2*pi/3) 0; 0 0 1]  Multiplication=Matrix(K*u)
  Gain1 : Gain  Gain=[exp(1i*2*pi/3) 0 0; 0 exp(1i*4*pi/3) 0; 0 0 1]  Multiplication=Matrix(K*u)
  Gain2 : Gain  Gain=180/pi
  Gain3 : Gain  Gain=180/pi
  Gain4 : Gain  Gain=180/pi
  Symmetrical-Components Transform1 : eeTransforms/Symmetrical-Components Transform  PowerInvariant=off
  ABC+-0 : Outport
  wires:
  Gain4/1 -> Demux5/1
  Gain3/1 -> Demux3/1
  Gain2/1 -> Demux1/1
  Demux5/1 -> Bus Creator8/1  "pos"
  Demux5/3 -> Bus Creator8/3  "zero"
  Demux5/2 -> Bus Creator8/2  "neg"
  Demux4/1 -> Bus Creator7/1  "pos"
  Demux4/3 -> Bus Creator7/3  "zero"
  Demux4/2 -> Bus Creator7/2  "neg"
  Demux3/1 -> Bus Creator2/1  "pos"
  Demux3/3 -> Bus Creator2/3  "zero"
  Demux3/2 -> Bus Creator2/2  "neg"
  Demux2/1 -> Bus Creator1/1  "pos"
  Demux2/3 -> Bus Creator1/3  "zero"
  Demux2/2 -> Bus Creator1/2  "neg"
  Demux1/2 -> Bus Creator4/2  "neg"
  Demux1/3 -> Bus Creator4/3  "zero"
  Demux1/1 -> Bus Creator4/1  "pos"
  Bus Creator/1 -> ABC+-0/1
  Gain1/1 -> Complex to Magnitude-Angle2/1
  Bus Creator9/1 -> Bus Creator/3  "C"
  Bus Creator8/1 -> Bus Creator9/2  "phase"
  Complex to Magnitude-Angle2/1 -> Demux4/1
  Bus Creator7/1 -> Bus Creator9/1  "mag"
  Complex to Magnitude-Angle2/2 -> Gain4/1
  Gain/1 -> Complex to Magnitude-Angle1/1
  Complex to Magnitude-Angle1/2 -> Gain3/1
  Bus Creator1/1 -> Bus Creator6/1  "mag"
  Complex to Magnitude-Angle1/1 -> Demux2/1
  Bus Creator2/1 -> Bus Creator6/2  "phase"
  Bus Creator6/1 -> Bus Creator/2  "B"
  Bus Creator5/1 -> Bus Creator/1  "A"
  abc/1 -> Symmetrical-Components Transform1/1
  Bus Creator4/1 -> Bus Creator5/2  "phase"
  Complex to Magnitude-Angle3/1 -> Demux/1
  Bus Creator3/1 -> Bus Creator5/1  "mag"
  Demux/3 -> Bus Creator3/3  "zero"
  Symmetrical-Components Transform1/1 -> Gain1/1, Gain/1, Complex to Magnitude-Angle3/1
  Demux/1 -> Bus Creator3/1  "pos"
  Complex to Magnitude-Angle3/2 -> Gain2/1
  Demux/2 -> Bus Creator3/2  "neg"

== system GridFormingConverter/Grid-Forming Converter/Controllers/Active Power Regulator (Preg) ==
  note: Active Power Regulator
  Pmeas : Inport  PortDimensions=1
  Pref : Inport  Port=2  PortDimensions=1  SampleTime=ConvCtrl.Ts
  On : Inport  Port=3  PortDimensions=1  SampleTime=ConvCtrl.Ts
  Discrete-Time Integrator : DiscreteIntegrator  InitialCondition=1  SampleTime=ConvCtrl.Ts  LimitOutput=on  UpperSaturationLimit=ConvCtrl.Preg.Limits(1)  LowerSaturationLimit=ConvCtrl.Preg.Limits(2)  ICPrevOutput=DiscIntNeverNeededParam  ICPrevScaledInput=DiscIntNeverNeededParam
  Product : Product  RndMeth=Zero
  Product1 : Product  RndMeth=Zero
  Product2 : Product
  Saturation2 : Saturate  UpperLimit=ConvCtrl.Preg.Limits(1)  LowerLimit=ConvCtrl.Preg.Limits(2)  SampleTime=ConvCtrl.Ts
  Sum : Sum  Inputs=|+-
  Sum6 : Sum  InputSameDT=on  SaturateOnIntegerOverflow=on  SampleTime=ConvCtrl.Ts  OutDataTypeStr=Inherit: Same as first input
  Switch1 : Switch  Criteria=u2 ~= 0  Threshold=0.5  OutDataTypeStr=double  SaturateOnIntegerOverflow=off  InputSameDT=off
  VdcNom_SM : Constant  Value=ConvCtrl.Preg.Kp  SampleTime=ConvCtrl.Ts
  VdcNom_SM1 : Constant  Value=ConvCtrl.Preg.Ki  SampleTime=ConvCtrl.Ts
  VdcNom_SM2 : Constant  Value=ConvPlt.Vnom_dc  SampleTime=ConvCtrl.Ts
  Zero-Order Hold : ZeroOrderHold  SampleTime=ConvCtrl.Ts
  Vdc_ref : Outport  SampleTime=ConvCtrl.Ts
  wires:
  Sum/1 -> Product/2, Product1/2
  Saturation2/1 -> Product2/1
  VdcNom_SM/1 -> Product1/1
  Product/1 -> Discrete-Time Integrator/1
  Product1/1 -> Zero-Order Hold/1
  VdcNom_SM1/1 -> Product/1
  Sum6/1 -> Saturation2/1
  Discrete-Time Integrator/1 -> Sum6/2
  Zero-Order Hold/1 -> Sum6/1
  Pref/1 -> Sum/2, Switch1/3
  Switch1/1 -> Sum/1
  On/1 -> Switch1/2
  Pmeas/1 -> Switch1/1
  VdcNom_SM2/1 -> Product2/2
  Product2/1 -> Vdc_ref/1

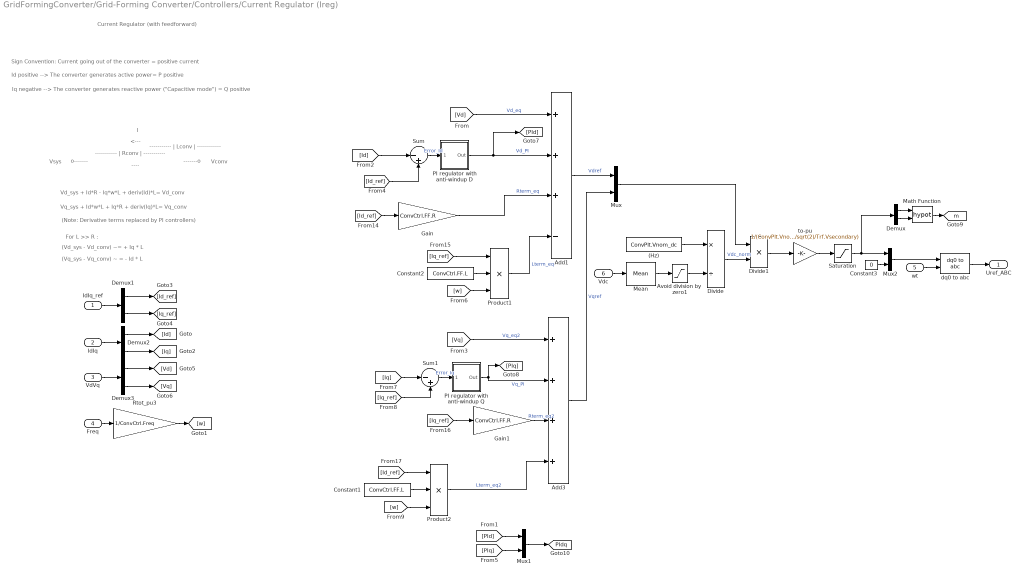
== system GridFormingConverter/Grid-Forming Converter/Controllers/Current Regulator (Ireg) ==
  note: I
  note: o-------
  note: Vsys
  note: (Note: Derivative terms replaced by PI controllers)
  note: Vd_sys + Id*R - Iq*w*L + deriv(Id)*L= Vd_conv
  note: Vq_sys + Id*w*L + Iq*R + deriv(Iq)*L= Vq_conv
  note: Current Regulator
      | (with feedforward)
  note: Sign Convention: Current going out of the converter = positive current
  note: Iq negative --> The converter generates reactive power ("Capacitive mode") = Q positive
  note: Id positive --> The converter generates active power= P positive
  note: (Vd_sys - Vd_conv) ~= + Iq * L
  note: (Vq_sys - Vq_conv) ~ = - Id * L
  note: For L >> R :
  note: -----------
      | | Rconv |
      | -----------
  note: ----
  note: Vconv
  note: -------o
  note: <---
  note: -----------
      | | Lconv |
      | ------------
  IdIq_ref : Inport  PortDimensions=2
  IdIq : Inport  Port=2  PortDimensions=2
  VdVq : Inport  Port=3  PortDimensions=2
  Freq : Inport  Port=4  PortDimensions=1
  wt : Inport  Port=5  PortDimensions=1
  Vdc : Inport  Port=6  PortDimensions=1
  " (Hz)" : Constant  Value=ConvPlt.Vnom_dc  SampleTime=ConvCtrl.Ts
  Add1 : Sum  Inputs=+++-
  Add3 : Sum  Inputs=++++
  Avoid division by zero1 : Saturate  UpperLimit=ConvPlt.Vnom_dc*1.25  LowerLimit=ConvPlt.Vnom_dc*0.75
  Constant1 : Constant  Value=ConvCtrl.FF.L  SampleTime=ConvCtrl.Ts
  Constant2 : Constant  Value=ConvCtrl.FF.L  SampleTime=ConvCtrl.Ts
  Constant3 : Constant  Value=0  SampleTime=ConvCtrl.Ts
  Demux{,1..3} (4 alike) : Demux  Outputs=2
  Divide : Product  Inputs=*/
  Divide1 : Product  Inputs=**
  Gain : Gain  Gain=ConvCtrl.FF.R
  Gain1 : Gain  Gain=ConvCtrl.FF.R
  Math Function : Math  Operator=hypot  SignedPower=on
  Mean : spsMeanLib/Mean  Freq=ConvCtrl.Freq/3  Vinit=ConvPlt.Vnom_dc  Ts=ConvCtrl.Ts
  Mux : Mux  Inputs=2
  Mux1 : Mux  Inputs=2
  Mux2 : Mux  Inputs=[2 1]
  PI regulator with anti-windup D : Subsystem  DialogController=POWERSYS.PowerSysDialog  mask(Discrete PI Controller){Kp=ConvCtrl.Ireg.Kp, Ki=ConvCtrl.Ireg.Ki, Par_Limits=ConvCtrl.Ireg.Limits, Init=0, Ts=ConvCtrl.Ts}
      mask prompts: Kp "Proportional gain (Kp):"; Ki "Integral gain (Ki):"; Par_Limits "Output limits: [ Upper   Lower ]"; Init "Output initial value:"; Ts "Sample time:"
      mask help: This block implements a discrete PI controller.
      mask init:
      | UpperLimit=Par_Limits(1);
      | LowerLimit=Par_Limits(2);
      | power_initmask();
      mask Help: This block is part of a subset of blocks in the Extras library that does not have documentation associated with it, other than the block mask description.
      mask Display: disp('PI');
  PI regulator with anti-windup Q : Subsystem  DialogController=POWERSYS.PowerSysDialog  mask(Discrete PI Controller){Kp=ConvCtrl.Ireg.Kp, Ki=ConvCtrl.Ireg.Ki, Par_Limits=ConvCtrl.Ireg.Limits, Init=0, Ts=ConvCtrl.Ts}
      mask prompts: Kp "Proportional gain (Kp):"; Ki "Integral gain (Ki):"; Par_Limits "Output limits: [ Upper   Lower ]"; Init "Output initial value:"; Ts "Sample time:"
      mask help: This block implements a discrete PI controller.
      mask init:
      | UpperLimit=Par_Limits(1);
      | LowerLimit=Par_Limits(2);
      | power_initmask();
      mask Help: This block is part of a subset of blocks in the Extras library that does not have documentation associated with it, other than the block mask description.
      mask Display: disp('PI');
  Product1 : Product  Inputs=3  RndMeth=Zero
  Product2 : Product  Inputs=3  RndMeth=Zero
  Rtot_pu3 : Gain  Gain=1/ConvCtrl.Freq  SaturateOnIntegerOverflow=on  OutDataTypeStr=Inherit: Same as input  ParamDataTypeStr=Inherit: Same as input
  Saturation : Saturate  UpperLimit=ConvCtrl.Ireg.Limits(1)  LowerLimit=ConvCtrl.Ireg.Limits(2)
  Sum : Sum  Inputs=|-+
  Sum1 : Sum  Inputs=|-+
  dq0 to abc : spsdq0toabcLib/dq0 to abc  Alignment=90 degrees behind phase A axis
  to-pu : Gain  Gain=1/(ConvPlt.Vnom_dc/2*sqrt(3)/sqrt(2)/Trf.Vsecondary)
  Uref_ABC : Outport
  tag scope: PIdq=global, m=global
  wires:
  Add3/1 -> Mux/2  "Vqref"
  Add1/1 -> Mux/1  "Vdref"
  Freq/1 -> Rtot_pu3/1
  Rtot_pu3/1 -> [w]
  Demux1/1 -> [Id_ref]
  Demux1/2 -> [Iq_ref]
  IdIq_ref/1 -> Demux1/1
  Demux3/1 -> [Vd]
  Demux3/2 -> [Vq]
  VdVq/1 -> Demux3/1
  Sum/1 -> PI regulator with anti-windup D/1(Error)  "Error_Id"
  [Id_ref] -> Sum/2
  Sum1/1 -> PI regulator with anti-windup Q/1(Error)  "Error_Iq"
  [Iq_ref] -> Sum1/2
  Constant1/1 -> Product2/2
  [w] -> Product2/3
  Constant2/1 -> Product1/2
  [w] -> Product1/3
  [PId] -> Mux1/1
  [PIq] -> Mux1/2
  Demux2/2 -> [Iq]
  [Iq] -> Sum1/1
  [Id] -> Sum/1
  [Id_ref] -> Gain/1
  [Iq_ref] -> Product1/1
  [Iq_ref] -> Gain1/1
  [Id_ref] -> Product2/1
  IdIq/1 -> Demux2/1
  Demux2/1 -> [Id]
  [Vq] -> Add3/1  "Vq_eq2"
  Product2/1 -> Add3/4  "Lterm_eq2"
  Gain1/1 -> Add3/3  "Rterm_eq2"
  Gain/1 -> Add1/3  "Rterm_eq"
  Product1/1 -> Add1/4  "Lterm_eq"
  [Vd] -> Add1/1  "Vd_eq"
  PI regulator with anti-windup Q/1(Out) -> Add3/2, [PIq]  "Vq_PI"
  PI regulator with anti-windup D/1(Out) -> Add1/2, [PId]  "Vd_PI"
  Saturation/1 -> Demux/1, Mux2/1
  Math Function/1 -> [m]
  Demux/1 -> Math Function/1
  Demux/2 -> Math Function/2
  Mux2/1 -> dq0 to abc/1
  Constant3/1 -> Mux2/2
  Mux1/1 -> [PIdq]
  Avoid division by zero1/1 -> Divide/2
  Vdc/1 -> Mean/1
  " (Hz)"/1 -> Divide/1
  Divide1/1 -> to-pu/1
  Mean/1 -> Avoid division by zero1/1
  Divide/1 -> Divide1/2  "Vdc_norm"
  dq0 to abc/1 -> Uref_ABC/1
  Mux/1 -> Divide1/1
  to-pu/1 -> Saturation/1
  wt/1 -> dq0 to abc/2

== system GridFormingConverter/Grid-Forming Converter/Controllers/DC Voltage Regulator (VDCreg) ==
  note: VDC Regulator
  Vdc_meas : Inport  PortDimensions=1
  Vdc_ref : Inport  Port=2  PortDimensions=1
  On : Inport  Port=3  PortDimensions=1
  Discrete-Time Integrator : DiscreteIntegrator  SampleTime=ConvCtrl.Ts  LimitOutput=on  UpperSaturationLimit=ConvCtrl.VDCreg.Limits(1)  LowerSaturationLimit=ConvCtrl.VDCreg.Limits(2)  ICPrevOutput=DiscIntNeverNeededParam  ICPrevScaledInput=DiscIntNeverNeededParam
  Product : Product  RndMeth=Zero
  Product1 : Product  RndMeth=Zero
  Rtot_pu2 : Gain  Gain=1/ConvPlt.Vnom_dc  SaturateOnIntegerOverflow=on  OutDataTypeStr=Inherit: Same as input  ParamDataTypeStr=Inherit: Same as input
  Saturation2 : Saturate  UpperLimit=ConvCtrl.VDCreg.Limits(1)  LowerLimit=ConvCtrl.VDCreg.Limits(2)  SampleTime=ConvCtrl.Ts
  Sum : Sum  Inputs=|+-
  Sum6 : Sum  InputSameDT=on  SaturateOnIntegerOverflow=on  SampleTime=ConvCtrl.Ts  OutDataTypeStr=Inherit: Same as first input
  Switch1 : Switch  Criteria=u2 ~= 0  Threshold=0.5  OutDataTypeStr=double  SaturateOnIntegerOverflow=off  InputSameDT=off
  VdcNom_SM : Constant  Value=ConvCtrl.VDCreg.Kp
  VdcNom_SM1 : Constant  Value=ConvCtrl.VDCreg.Ki
  Zero-Order Hold : ZeroOrderHold  SampleTime=ConvCtrl.Ts
  Id_ref : Outport
  wires:
  Vdc_meas/1 -> Switch1/1
  Sum/1 -> Rtot_pu2/1
  On/1 -> Switch1/2
  Switch1/1 -> Sum/1
  Vdc_ref/1 -> Switch1/3, Sum/2
  Zero-Order Hold/1 -> Sum6/1
  Discrete-Time Integrator/1 -> Sum6/2
  Sum6/1 -> Saturation2/1
  VdcNom_SM1/1 -> Product/1
  Product1/1 -> Zero-Order Hold/1
  Product/1 -> Discrete-Time Integrator/1
  VdcNom_SM/1 -> Product1/1
  Saturation2/1 -> Id_ref/1
  Rtot_pu2/1 -> Product1/2, Product/2

== system GridFormingConverter/Grid-Forming Converter/Controllers/Mode of Operation Panel ==
  In1 : Inport
  Enable : EnablePort
  MATLAB Function (Mode of Operation - Converter 1) : MATLAB Function  TreatAsAtomicUnit=on
  wires:
  In1/1 -> MATLAB Function (Mode of Operation - Converter 1)/1(u)

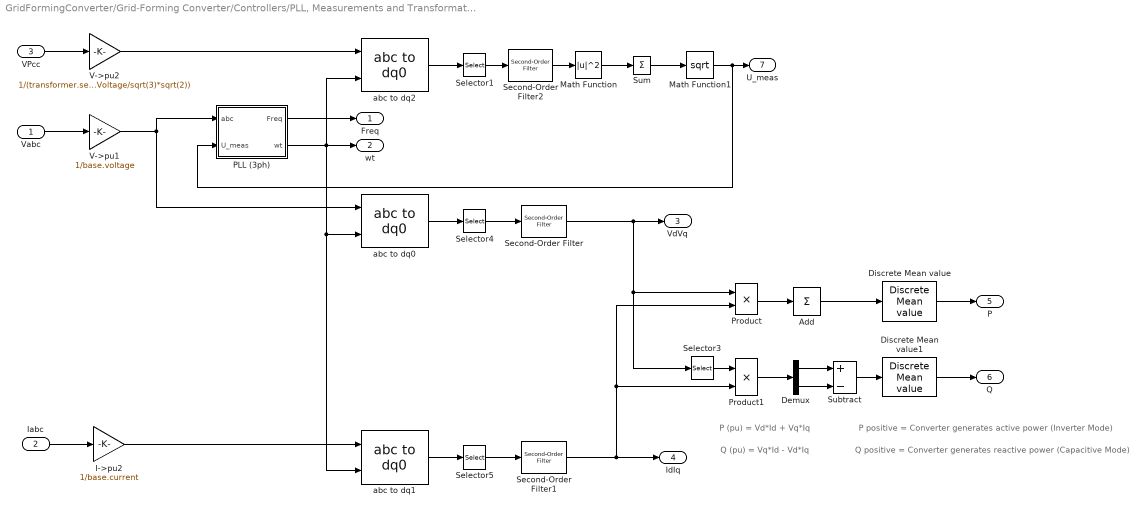
== system GridFormingConverter/Grid-Forming Converter/Controllers/PLL, Measurements and Transformation ==
  note: Q positive = Converter generates reactive power (Capacitive Mode)
  note: P positive = Converter generates active power (Inverter Mode)
  note: Q (pu) = Vq*Id - Vd*Iq
  note: P (pu) = Vd*Id + Vq*Iq
  Vabc : Inport  PortDimensions=3
  Iabc : Inport  Port=2  PortDimensions=3
  VPcc : Inport  Port=3
  Add : Sum  Inputs=1
  Demux : Demux  Outputs=2
  Discrete Mean value : powerlib_extras/Discrete Measurements/Discrete  Mean value  Freq=ConvCtrl.Freq  Vinit=0  Ts=ConvCtrl.Ts
  Discrete Mean value1 : powerlib_extras/Discrete Measurements/Discrete  Mean value  Freq=ConvCtrl.Freq  Vinit=0  Ts=ConvCtrl.Ts
  I->pu2 : Gain  Gain=1/base.current  SaturateOnIntegerOverflow=on  OutDataTypeStr=Inherit: Same as input  ParamDataTypeStr=Inherit: Same as input
  Math Function : Math  Operator=magnitude^2  SignedPower=on
  Math Function1 : Math  Operator=sqrt  SignedPower=on
  PLL (3ph) : Subsystem  AncestorBlock=|  DialogController=POWERSYS.PowerSysDialog  LoadFcn=sps_rtmsupport('LoadFcn', gcbh);  StartFcn=sps_rtmsupport('StartFcn', gcbh);  StopFcn=sps_rtmsupport('StopFcn', gcbh);  mask(PLL (3ph)){Fmin=ConvCtrl.PLL.MinFreq, Par_Init=[0, ConvCtrl.PLL.InitFreq], ParK=[ConvCtrl.PLL.Kp, ConvCtrl.PLL.Ki, ConvCtrl.PLL.Kd], TcD=ConvCtrl.PLL.Ts, MaxRateChangeFreq=ConvCtrl.PLL.MaxRocof, FilterCutOffFreq=ConvCtrl.PLL.Fc_filter, Ts=ConvCtrl.Ts, AGC=on}
      | sps_lib/Control/PLL
      | (3ph)
      mask prompts: Fmin "Minimum frequency (Hz):"; Par_Init "Initial inputs [ Phase (degrees), Frequency (Hz) ]:"; ParK "Regulator gains [ Kp, Ki, Kd ]:"; TcD "Time constant for derivative action (s):"; MaxRateChangeFreq "Maximum rate of change of frequency (Hz/s):"; FilterCutOffFreq "Filter cut-off frequency for frequency measurement (Hz):"; Ts "Sample time:"; AGC "Enable automatic gain control"
      mask help:
      | This Phase Locked Loop (PLL) system can be used  to synchronize on a set of variable frequency, three-phase sinusoidal signals. If the Automatic Gain Control is enabled, the input (phase error) of the PLL regulator is scaled according to the input signals magnitude.
      |
      | For optimal performance, set regulator gains [ Kp Ki  Kd ] = [ 180  3200  1 ] and check the Enable Automatic Gain Control parameter.
      |
      | Input : Vector containing the normalized three-phase signals [Va Vb Vc]
      | Output 1:  Measured frequency (Hz) = w/(2pi)
      | Output 2:  Ramp w.t varying between  0 and 2*pi, synchronized on zero crossings of the fundamental (positive-sequence) of phase A.
      mask init:
      | block=gcb;
      | [WantBlockChoice,Ts,sps] = powericon('PLL3phInit',block,Fmin,Par_Init,ParK,TcD, MaxRateChangeFreq, FilterCutOffFreq, AGC,Ts);
      | powericon('SetInternalModels','set',block,WantBlockChoice);
      settings: CopyFcn=sps_rtmsupport('CopyFcn', gcbh);  DeleteFcn=sps_rtmsupport('DeleteFcn', gcbh);  UndoDeleteFcn=sps_rtmsupport('UndoDeleteFcn', gcbh);  ModelCloseFcn=sps_rtmsupport('ModelCloseFcn', gcbh);  PreSaveFcn=sps_rtmsupport('PreSaveFcn', gcbh);  PostSaveFcn=sps_rtmsupport('PostSaveFcn', gcbh);  NameChangeFcn=sps_rtmsupport('NameChangeFcn', gcbh);  PreCopyFcn=sps_rtmsupport('PreCopyFcn', gcbh);  OpenFcn=sps_rtmsupport('OpenFcn', gcbh, [8]);  CloseFcn=sps_rtmsupport('CloseFcn', gcbh);  PreDeleteFcn=sps_rtmsupport('PreDeleteFcn', gcbh);
      settings: LibrarySourceBlock=|
      | sps_lib/Control/PLL
      | (3ph)
      mask Help: helpview(psbhelp);
  Product : Product  RndMeth=Zero
  Product1 : Product  RndMeth=Zero
  Second-Order Filter : spsSecondOrderFilterLib/Second-Order Filter  FilterType=Lowpass  Fo=ConvCtrl.Fn_filter  Zeta=ConvCtrl.Zeta_filter  Ts=ConvCtrl.Ts  Initialize=off  Vac_Init="[0,  0,  60]"  Vdc_Init=0  PlotResponse=off  FreqRange=[0, 500, 1]
      settings: LibrarySourceBlock=|
      | sps_lib/Control/Filters/Second-Order
      | Filter
  Second-Order Filter1 : spsSecondOrderFilterLib/Second-Order Filter  FilterType=Lowpass  Fo=ConvCtrl.Fn_filter  Zeta=ConvCtrl.Zeta_filter  Ts=ConvCtrl.Ts  Initialize=off  Vac_Init="[0,  0,  60]"  Vdc_Init=0  PlotResponse=off  FreqRange=[0, 500, 1]
      settings: LibrarySourceBlock=|
      | sps_lib/Control/Filters/Second-Order
      | Filter
  Second-Order Filter2 : spsSecondOrderFilterLib/Second-Order Filter  FilterType=Lowpass  Fo=ConvCtrl.Fn_filter  Zeta=ConvCtrl.Zeta_filter  Ts=ConvCtrl.Ts  Initialize=off  Vac_Init="[0,  0,  60]"  Vdc_Init=0  PlotResponse=off  FreqRange=[0, 500, 1]
      settings: LibrarySourceBlock=|
      | sps_lib/Control/Filters/Second-Order
      | Filter
  Selector1 : Selector  InputPortWidth=3  IndexOptions=Index vector (dialog)  Indices=[1 2]  OutputSizes=1
  Selector3 : Selector  InputPortWidth=2  IndexOptions=Index vector (dialog)  Indices=[2 1]  OutputSizes=1
  Selector4 : Selector  InputPortWidth=3  IndexOptions=Index vector (dialog)  Indices=[1 2]  OutputSizes=1
  Selector5 : Selector  InputPortWidth=3  IndexOptions=Index vector (dialog)  Indices=[1 2]  OutputSizes=1
  Subtract : Sum  Inputs=+-
  Sum : Sum  Inputs=+  SaturateOnIntegerOverflow=on
  V->pu1 : Gain  Gain=1/base.voltage  SaturateOnIntegerOverflow=on  OutDataTypeStr=Inherit: Same as input  ParamDataTypeStr=Inherit: Same as input
  V->pu2 : Gain  Gain=1/(transformer.secondaryRMSVoltage/sqrt(3)*sqrt(2))  SaturateOnIntegerOverflow=on  OutDataTypeStr=Inherit: Same as input  ParamDataTypeStr=Inherit: Same as input
  abc to dq0 : spsabctodq0Lib/abc to dq0  Alignment=90 degrees behind phase A axis
  abc to dq1 : spsabctodq0Lib/abc to dq0  Alignment=90 degrees behind phase A axis
  abc to dq2 : spsabctodq0Lib/abc to dq0  Alignment=90 degrees behind phase A axis
  Freq : Outport
  wt : Outport  Port=2
  VdVq : Outport  Port=3
  IdIq : Outport  Port=4
  P : Outport  Port=5
  Q : Outport  Port=6
  U_meas : Outport  Port=7  VectorParamsAs1DForOutWhenUnconnected=off
  wires:
  Math Function1/1 -> PLL (3ph)/2(U_meas), U_meas/1
  Second-Order Filter2/1 -> Math Function/1
  Sum/1 -> Math Function1/1
  Math Function/1 -> Sum/1
  Selector1/1 -> Second-Order Filter2/1
  abc to dq2/1 -> Selector1/1
  V->pu2/1 -> abc to dq2/1
  VPcc/1 -> V->pu2/1
  Selector5/1 -> Second-Order Filter1/1
  Selector4/1 -> Second-Order Filter/1
  I->pu2/1 -> abc to dq1/1
  abc to dq1/1 -> Selector5/1
  Iabc/1 -> I->pu2/1
  PLL (3ph)/2(wt) -> abc to dq0/2, abc to dq1/2, abc to dq2/2, wt/1
  Vabc/1 -> V->pu1/1
  V->pu1/1 -> PLL (3ph)/1(abc), abc to dq0/1
  PLL (3ph)/1(Freq) -> Freq/1
  abc to dq0/1 -> Selector4/1
  Subtract/1 -> Discrete Mean value1/1
  Add/1 -> Discrete Mean value/1
  Demux/2 -> Subtract/2
  Demux/1 -> Subtract/1
  Product1/1 -> Demux/1
  Product/1 -> Add/1
  Second-Order Filter1/1 -> Product/2, Product1/2, IdIq/1
  Discrete Mean value/1 -> P/1
  Discrete Mean value1/1 -> Q/1
  Selector3/1 -> Product1/1
  Second-Order Filter/1 -> Selector3/1, Product/1, VdVq/1
